simulink model "PI_controller"  (R2020b)
settings: Solver=VariableStepAuto  StartTime=0.0  StopTime=10.0  RelTol=1e-3
values from neighbouring files (symbols this model uses):
  ki = 40    [values.m]
  kp = 800    [values.m]
  ts = 1    [values.m]
settings Model: Creator=Abhinav dixit  LastModifiedBy=Abhinav dixit
settings DataIOCC: SaveOutput=off  SaveTime=off

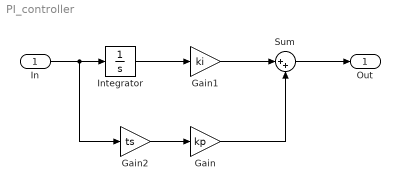
== system PI_controller ==
  In : Inport  OutDataTypeStr=double  PortDimensions=1  SampleTime=0
  Gain : Gain  Gain=kp
  Gain1 : Gain  Gain=ki
  Gain2 : Gain  Gain=ts
  Integrator : Integrator
  Sum : Sum  Inputs=|++
  Out : Outport  OutDataTypeStr=double  PortDimensions=1  SampleTime=0
  wires:
  Integrator/1 -> Gain1/1
  In/1 -> Integrator/1, Gain2/1
  Gain1/1 -> Sum/1
  Gain/1 -> Sum/2
  Sum/1 -> Out/1
  Gain2/1 -> Gain/1
